simulink model "Final_simu"  (R2023a)
settings: Solver=FixedStepAuto  StartTime=0.0  StopTime=10  RelTol=1e-3
undefined symbols (not defined in the file): Kalpha, Kbeta, Krho, theta_a, thetastar, x_a, xstar, y_a, ystar
settings Model: Creator=daneydem1u  LastModifiedBy=daneydem1u

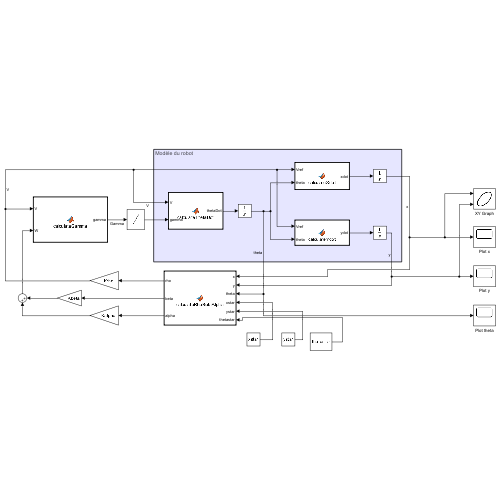
[thumbnail: Simulink's stored preview of the top-level diagram]
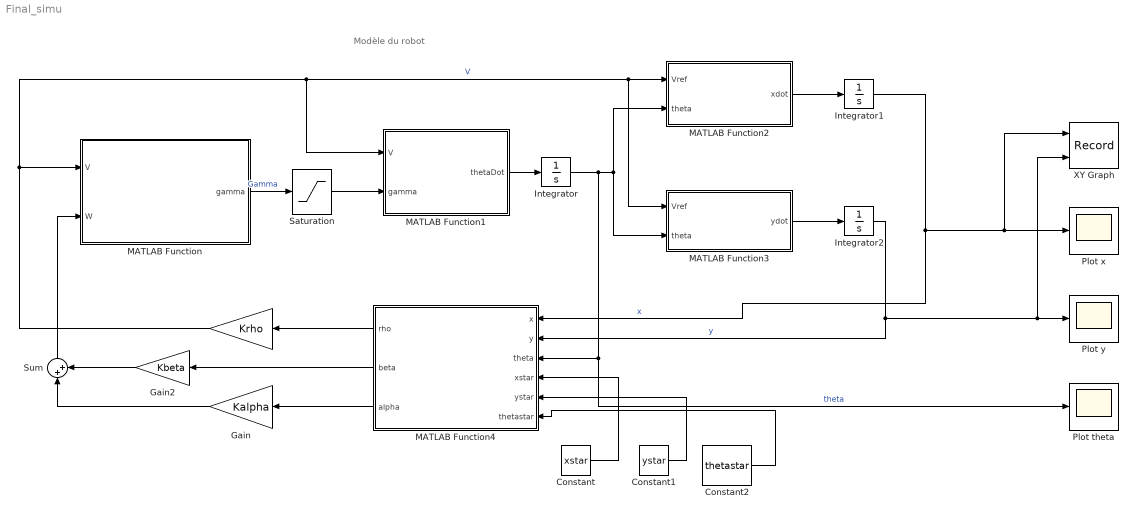
== system Final_simu ==
  note: Modèle du robot
  " " : Gain  Gain=Krho
  Constant : Constant  Value=xstar
  Constant1 : Constant  Value=ystar
  Constant2 : Constant  Value=thetastar
  Gain : Gain  Gain=Kalpha
  Gain2 : Gain  Gain=Kbeta
  Integrator : Integrator  InitialCondition=theta_a
  Integrator1 : Integrator  InitialCondition=x_a
  Integrator2 : Integrator  InitialCondition=y_a
  MATLAB Function : MATLAB Function  TreatAsAtomicUnit=on
  MATLAB Function1 : MATLAB Function  TreatAsAtomicUnit=on
  MATLAB Function2 : MATLAB Function  TreatAsAtomicUnit=on
  MATLAB Function3 : MATLAB Function  TreatAsAtomicUnit=on
  MATLAB Function4 : MATLAB Function  TreatAsAtomicUnit=on
  Plot theta : Scope
  Plot x : Scope
  Plot y : Scope
  Saturation : Saturate  UpperLimit=pi/2  LowerLimit=-pi/2
  Sum : Sum  Inputs=|++
  XY Graph : Record  FileSettingsInternal="{\"entries\":[{\"content\":{\"excelSettings\":{\"content\":{},\"type\":\"Streamout.ExcelSettings\"}},\"type\":\"Streamout.FileSettingStorage\",\"uuid\":\"2f5fa65a-796f-4f7d-891b-f8713251b2e0\"}],\"packageUris\":[\"http://schema.mathworks.com/mf0/streamout_blocks/R2020a\"],\"version\":\"1.0\"}"  Layout=[1 1]  SignalsInternal="{\"entries\":[{\"content\":{\"signals\":[{\"content\":{\"blockPath\":[\"Final_simu/XY Graph\"],\"dimensions\":[1],\"domain\":\"Final_simu/XY Graph\",\"lineColor\":\"#a2142f\",\"plots\":[1],\"port\":1,\"sid\":[\"\"],\"signalID\":291,\"signalName\":\"x\"},\"type\":\"RecordBlkView.Signal\",\"uuid\":\"d41bd4e5-6e78-4546-b62c-79ccecbda96c\"},{\"content\":{\"blockPath\":[\"Final_simu/XY Graph\"],\"dimensions\":[1],\"domain\":\"Final_simu/XY Graph\",\"lineColor\":\"#139fff\",\"plots\":[1],\"port\":2,\"sid\":[\"\"],\"signalID\":295,\"signalName\":\"y\"},\"type\":\"RecordBlkView.Signal\",\"uuid\":\"ffe9e9b2-156e-4968-97ea-6afee1f50c1e\"}]},\"type\":\"RecordBlkView.InputSignals\",\"uuid\":\"cdfb4a85-8cfa-4561-8577-a7b2b6cd829f\"}],\"packageUris\":[\"http://schema.mathworks.com/mf0/streamout_blocks/R2020a\"],\"version\":\"1.0\"}"  VisualizationBindings="{\"xyplotplugin\":{\"info\":[{\"series\":[{\"bindingParametersList\":[{\"parameter\":\"X-Axis\",\"signalID\":291,\"signalName\":\"x\"},{\"parameter\":\"Y-Axis\",\"signalID\":295,\"signalName\":\"y\"}],\"seriesID\":39630}],\"subplotID\":1}]}}"  CompatibilityTag=XY
  wires:
  " "/1 -> MATLAB Function/1(V), MATLAB Function1/1(V), MATLAB Function3/1(Vref), MATLAB Function2/1(Vref)  "V"
  Sum/1 -> MATLAB Function/2(W)
  MATLAB Function1/1(thetaDot) -> Integrator/1
  Integrator/1 -> Plot theta/1, MATLAB Function4/3(theta), MATLAB Function2/2(theta), MATLAB Function3/2(theta)  "theta"
  MATLAB Function2/1(xdot) -> Integrator1/1
  MATLAB Function3/1(ydot) -> Integrator2/1
  Integrator1/1 -> MATLAB Function4/1(x), XY Graph/1, Plot x/1  "x"
  Integrator2/1 -> MATLAB Function4/2(y), XY Graph/2, Plot y/1  "y"
  MATLAB Function4/1(rho) -> " "/1
  MATLAB Function4/2(beta) -> Gain2/1
  MATLAB Function4/3(alpha) -> Gain/1
  Gain2/1 -> Sum/2
  Gain/1 -> Sum/1
  Saturation/1 -> MATLAB Function1/2(gamma)
  MATLAB Function/1(gamma) -> Saturation/1  "Gamma"
  Constant/1 -> MATLAB Function4/4(xstar)
  Constant1/1 -> MATLAB Function4/5(ystar)
  Constant2/1 -> MATLAB Function4/6(thetastar)

== matlab function Final_simu/MATLAB Function1 ==
  data: V input; thetaDot output; gamma input; longueur parameter
function thetaDot = calculateThetaDot(V, gamma, longueur)
    % Calcul de thetaDot
    thetaDot = V * tan(gamma) / longueur;
end

== matlab function Final_simu/MATLAB Function ==
  data: V input; gamma output; W input; longueur parameter
function gamma = calculateGamma(V, W, longueur)
    gamma = atan((W * longueur) / V);
end

== matlab function Final_simu/MATLAB Function2 ==
  data: Vref input; xdot output; theta input
function xdot = calculateXdot(Vref, theta)
    xdot = Vref * cos(theta);
end

== matlab function Final_simu/MATLAB Function3 ==
  data: Vref input; ydot output; theta input
function ydot = calculateYdot(Vref, theta)
    ydot = Vref * sin(theta);
end

== matlab function Final_simu/MATLAB Function4 ==
  data: x input; rho output; y input; theta input; beta output; alpha output; xstar input; ystar input; thetastar input
function [rho, beta, alpha] = calculateRhoBetaAlpha(x, y, theta, xstar, ystar, thetastar)
    dx = xstar - x;
    dy = ystar - y;

    rho = sqrt(dx^2 + dy^2); % Distance euclidienne à la cible

    % Calcul de l'angle alpha
    alpha_to_target = atan2(dy, dx); 
    alpha = wrapToPi(alpha_to_target - theta); 

    % Calcul de l'angle beta
    beta = wrapToPi(thetastar - theta); 
end
